simulink model "puissance_exo"  (R2024b)
settings: Solver=VariableStepAuto  StartTime=0.0  StopTime=10.0  RelTol=1e-3
values from neighbouring files (symbols this model uses):
  Tf = 0.2    [defvars.m]
libraries: simulink x2
settings Model: Creator=marc.nicoller  LastModifiedBy=marc.nicoller

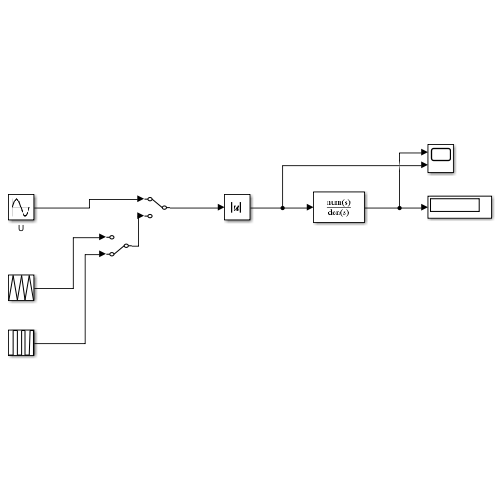
[thumbnail: Simulink's stored preview of the top-level diagram]
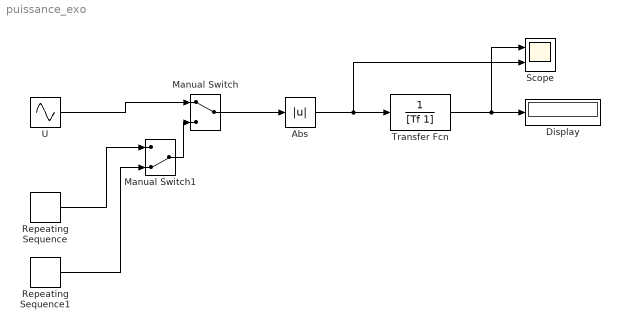
== system puissance_exo ==
  Abs : Abs  SaturateOnIntegerOverflow=off
  Display : Display
  Manual Switch : ManualSwitch
  Manual Switch1 : ManualSwitch  CurrentSetting=0
  Repeating Sequence : simulink/Sources/Repeating Sequence  rep_seq_t=[0 0.01 0.02]  rep_seq_y=[-1 1 -1]
  Repeating Sequence1 : simulink/Sources/Repeating Sequence  rep_seq_t=[0 0.01 0.011 0.02]  rep_seq_y=[-1 -1 1 1]
  Scope : Scope  NumInputPorts=2
  Transfer Fcn : TransferFcn  Denominator=[Tf 1]
  U : Sin  Frequency=2*pi*50  SampleTime=0
  wires:
  Repeating Sequence/1 -> Manual Switch1/1
  Repeating Sequence1/1 -> Manual Switch1/2
  Abs/1 -> Scope/2, Transfer Fcn/1
  Manual Switch1/1 -> Manual Switch/2
  Transfer Fcn/1 -> Scope/1, Display/1
  U/1 -> Manual Switch/1
  Manual Switch/1 -> Abs/1
